simulink model "power_breaker"  (Simulink 6.0)
settings: Solver=ode23tb  SolverMode=SingleTasking  StartTime=0.0  StopTime=0.1  MaxStep=100e-6  RelTol=1e-3
libraries: powerlib x6, powerlib_extras x1
settings Model: Creator=patrice  LastModifiedBy=batserve  ExtModeTrigMode=oneshot  ExtModeArmWhenConnect=off  ExtModeAutoUpdateStatusClock=off
settings DataIOCC: LimitDataPoints=off  SignalLoggingName=sigsOut
settings OptimizationCC: BooleanDataType=off
settings DebuggingCC: SolverPrmCheckMsg=none
settings HardwareCC: TargetUnknown=on
settings RTWCC: TemplateMakefile=grt_unix.tmf

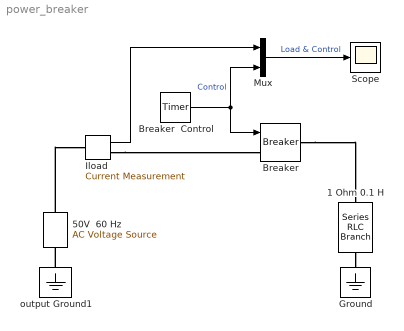
== system power_breaker ==
  1 Ohm 0.1 H : powerlib/Elements/Series RLC Branch  Orientation=down  PhysicalDomain=powersysdomain  SubClassName=unknown  PortType=p1  LConnTagsString=__new0  RConnTagsString=__new0  Resistance=1  Inductance=0.1  Capacitance=inf  Measurements=None
  50V  60 Hz : powerlib/Electrical Sources/AC Voltage Source  Description=source block  Orientation=up  Amplitude=50  Phase=0  Frequency=60  SampleTime=0  Measurements=None
      settings: AttributesFormatString=\n
  Breaker : powerlib/Elements/Breaker  BreakerResistance=1e-4  InitialState=1  SnubberResistance=1e6  SnubberCapacitance=inf  SwitchingTimes="[ 4/60  5/60 ]"  External=on  Measurements=None
      settings: AttributesFormatString=\n
  Breaker  Control : powerlib_extras/Control  Blocks/Timer  t=[0 1.5/60 3/60]  e=[1 0 1 ]
  Ground : powerlib/Elements/Ground  Orientation=down  PhysicalDomain=powersysdomain  SubClassName=unknown  PortType=p1  LConnTagsString=a
  Iload : powerlib/Measurements/Current Measurement  Tag=PoWeRsYsTeMmEaSuReMeNt  PhasorSimulation=off  OutputType=Magnitude  PSBequivalent=0
  Mux : Mux  Inputs=2
  Scope : Scope
      settings: TimeRange=0.1  YMin=-2  YMax=3  DataFormat=Array
  output Ground1 : powerlib/Elements/Ground  Orientation=down  PhysicalDomain=powersysdomain  SubClassName=unknown  PortType=p1  LConnTagsString=a
  wires:
  Mux/1 -> Scope/1  "Load & Control"
  Iload/1 -> Mux/1
  Breaker  Control/1 -> Breaker/1, Mux/2  "Control"
  connections:
  Iload/RConn1 -- Breaker/LConn1
  50V  60 Hz/RConn1 -- Iload/LConn1
  output Ground1/LConn1 -- 50V  60 Hz/LConn1
  1 Ohm 0.1 H/RConn1 -- Ground/LConn1
  Breaker/RConn1 -- 1 Ohm 0.1 H/LConn1
